simulink model "Y1_v2_v12"  (R2020a)
settings: Solver=VariableStepAuto  StartTime=0.0  StopTime=0.3  MaxStep=1e-5  RelTol=1e-3  EnableMultiTasking=on
libraries: simulink x1
settings Model: SimulationMode=accelerator  Creator=OXAALJ  LastModifiedBy=nxf75332
settings SolverCC: MaxOrder=2  MaxConsecutiveZCs=10  MaxConsecutiveMinStep=10  ZeroCrossControl=DisableAll
settings DataIOCC: LimitDataPoints=on  SaveFormat=Array  DSMLogging=off  ReturnWorkspaceOutputs=off
settings OptimizationCC: LifeSpan=inf
settings DebuggingCC: UnderspecifiedInitializationDetection=Classic  MergeDetectMultiDrivingBlocksExec=none  SolverPrmCheckMsg=warning  MultiTaskDSMMsg=warning  MultiTaskCondExecSysMsg=none  StateNameClashWarn=warning  SFUnexpectedBacktrackingDiag=warning  SFNoUnconditionalDefaultTransitionDiag=warning  SFExecutionAtInitializationDiag=none  ArithmeticOperatorsInVariantConditions=warning
settings HardwareCC: ProdBitPerPointer=32  ProdBitPerSizeT=32  ProdBitPerPtrDiffT=32  ProdLargestAtomicFloat=None  ProdIntDivRoundTo=Undefined  ProdEndianess=Unspecified  ProdWordSize=32  ProdHWDeviceType=32-bit Generic
settings ModelReferenceCC: PropagateSignalLabelsOutOfModel=off
settings SFSimCC: SimUseLocalCustomCode=off  CustomCodeUndefinedFunction=UseInterfaceOnly
settings RTWCC: RTWUseLocalCustomCode=off
settings CodeAppCC: StateflowObjectComments=on
settings GRTTargetCC: TargetLangStandard=C89/C90 (ANSI)
settings ConfigComp: CovMetricSettings=dw  CovHtmlReporting=on  CovSaveCumulativeToWorkspaceVar=on  CovSaveSingleToWorkspaceVar=on  CovExternalEMLEnable=off  CovSFcnEnable=off

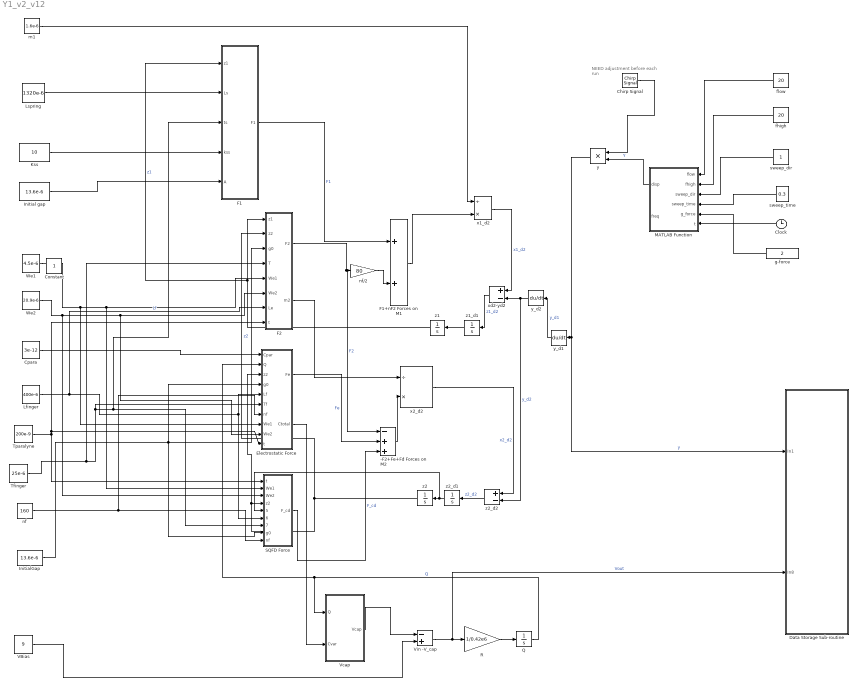
== system Y1_v2_v12 ==
  note: NEED
      | adjustment
      | before each
      | run
  -F2+Fe+Fd Forces on M2 : Sum  Inputs=-++  RndMeth=Nearest
  Chirp Signal : simulink/Sources/Chirp Signal  f1=20  T=0.3  f2=20
  Clock : Clock
  Cpara : Constant  Value=3e-12  VectorParams1D=off
  Data Storage Sub-routine : Subsystem
  Electrostatic Force : MATLAB Function  TreatAsAtomicUnit=on
  F1 : MATLAB Function  TreatAsAtomicUnit=on
  F1+nF2 Forces on M1 : Sum  RndMeth=Nearest
  F2 : MATLAB Function  TreatAsAtomicUnit=on
  Initial gap : Constant  Value=13.6e-6
  InitialGap : Constant  Value=13.6e-6
  Kss : Constant  Value=10
  Lfinger : Constant  Value=400e-6
  Lspring : Constant  Value=1320e-6
  MATLAB Function : MATLAB Function  TreatAsAtomicUnit=on
  Q : Integrator
  R : Gain  Gain=1/0.42e6
  SQFD Force : MATLAB Function  TreatAsAtomicUnit=on
  Tfinger : Constant  Value=25e-6
  Tparalyne : Constant  Value=200e-9  VectorParams1D=off
  VBias : Constant  Value=9
  Vcap : MATLAB Function  TreatAsAtomicUnit=on
  Vin -V_cap : Sum  Inputs=-+  RndMeth=Nearest
  We1 : Constant  Value=4.5e-6  VectorParams1D=off
  We2 : Constant  Value=20.9e-6  VectorParams1D=off
  fhigh : Constant  Value=20
  flow : Constant  Value=20
  g-force : Constant  Value=2
  m1 : Constant  Value=1.6e-6
  nf : Constant  Value=160
  nf/2 : Gain  Gain=80
  sweep_dir : Constant
  sweep_time : Constant  Value=0.3
  x1_d2 : Product  Inputs=/*
  x2_d2 : Product  Inputs=/*
  xd2-yd2 : Sum  Inputs=+-  RndMeth=Nearest
  y : Product
  y_d1 : Derivative
  y_d2 : Derivative
  z1 : Integrator
  z1_d1 : Integrator
  z2 : Integrator
  z2_d1 : Integrator
  z2_d2 : Sum  Inputs=+-  RndMeth=Nearest
  Constant : Constant  IOType=siggen
  wires:
  Electrostatic Force/1(Fe) -> -F2+Fe+Fd Forces on M2/2  "Fe"
  F1/1(F1) -> F1+nF2 Forces on M1/1  "F1"
  SQFD Force/1(F_cd) -> -F2+Fe+Fd Forces on M2/3  "F_cd"
  m1/1 -> x1_d2/1
  Clock/1 -> MATLAB Function/6(t)
  g-force/1 -> MATLAB Function/5(g_force)
  sweep_time/1 -> MATLAB Function/4(sweep_time)
  fhigh/1 -> MATLAB Function/2(fhigh)
  flow/1 -> MATLAB Function/1(flow)
  sweep_dir/1 -> MATLAB Function/3(sweep_dir)
  MATLAB Function/1(disp) -> y/2  "Y"
  y/1 -> Data Storage Sub-routine/1(In1), y_d1/1  "y"
  InitialGap/1 -> Electrostatic Force/4(g0), SQFD Force/8(g0), F2/3(g0)
  VBias/1 -> Vin -V_cap/2
  Vin -V_cap/1 -> Data Storage Sub-routine/2(In8), R/1  "Vout"
  R/1 -> Q/1
  Q/1 -> Electrostatic Force/2(Q), Vcap/1(Q)  "Q"
  Vcap/1(Vcap) -> Vin -V_cap/1
  Lfinger/1 -> F2/7(Le), Electrostatic Force/5(Lf), SQFD Force/6(Lf_damp)  "Lf"
  Cpara/1 -> Electrostatic Force/1(Cpar)
  Chirp Signal/1 -> y/1
  nf/1 -> Electrostatic Force/7(nf), SQFD Force/9(nf)
  Lspring/1 -> F1/2(Ls)
  Tfinger/1 -> F2/4(T), Electrostatic Force/6(Tf), F1/3(ts), SQFD Force/7(Tf_damp)
  Kss/1 -> F1/4(kss)
  F2/1(F2) -> -F2+Fe+Fd Forces on M2/1, nf/2/1  "F2"
  F1+nF2 Forces on M1/1 -> x1_d2/2
  y_d1/1 -> y_d2/1  "y_d1"
  x1_d2/1 -> xd2-yd2/1  "x1_d2"
  y_d2/1 -> z2_d2/2, xd2-yd2/2  "y_d2"
  xd2-yd2/1 -> z1_d1/1  "z1_d2"
  z1_d1/1 -> z1/1
  z1/1 -> F1/1(z1), F2/1(z1)  "z1"
  x2_d2/1 -> z2_d2/1  "x2_d2"
  z2_d2/1 -> z2_d1/1  "z2_d2"
  z2_d1/1 -> SQFD Force/5(z2_d1), z2/1
  z2/1 -> Electrostatic Force/3(z2), SQFD Force/4(z2), F2/2(z2)  "z2"
  F2/2(m2) -> x2_d2/1
  -F2+Fe+Fd Forces on M2/1 -> x2_d2/2
  nf/2/1 -> F1+nF2 Forces on M1/2
  Electrostatic Force/2(Ctotal) -> Vcap/2(Cvar)
  Initial gap/1 -> F1/5(A)
  We1/1 -> Electrostatic Force/8(We1), SQFD Force/2(We1), F2/5(We1)
  We2/1 -> SQFD Force/3(We2), Electrostatic Force/9(We2), F2/6(We2)
  Tparalyne/1 -> Electrostatic Force/10(t), F2/8(t), SQFD Force/1(t)

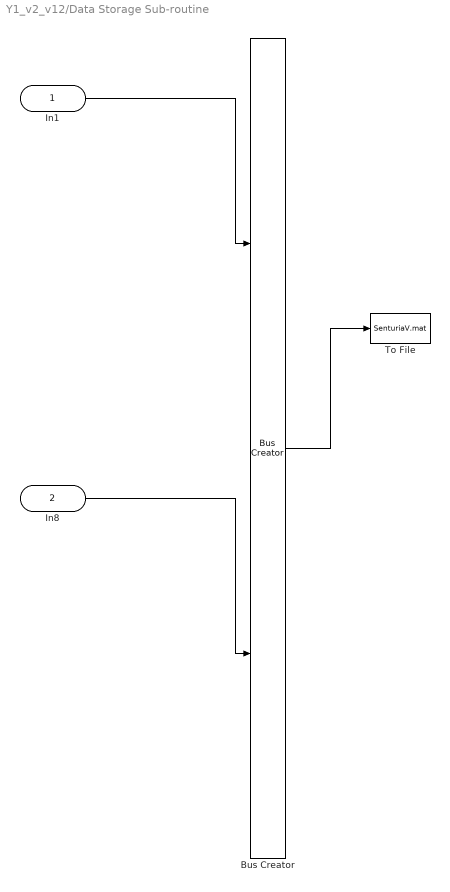
== system Y1_v2_v12/Data Storage Sub-routine ==
  In1 : Inport
  In8 : Inport  Port=2
  Bus Creator : BusCreator  Inputs=2
  To File : ToFile  Filename=SenturiaV.mat  SaveFormat=Timeseries
  wires:
  Bus Creator/1 -> To File/1
  In1/1 -> Bus Creator/1
  In8/1 -> Bus Creator/2

== matlab function Y1_v2_v12/Vcap ==
  data: Q input; Cvar input; Vcap output
function Vcap   = fcn(Q, Cvar)
Vcap = Q/Cvar;
end

== matlab function Y1_v2_v12/Electrostatic Force ==
  data: Cpar input; Q input; z2 input; g0 input; Lf input; Tf input; nf input; We1 input; Fe output; Ctotal output; We2 input; t input
function [Fe,Ctotal] = fcn(Cpar,Q,z2,g0,Lf,Tf,nf, We1, We2, t)
% This function is to calculate the Fe (electrostatic force on m2)

Lfeff =  Lf;
Tfeff =  Tf;
Lf    =  Tfeff;
Tf    =  Lfeff;


%%%% slanted electrodes (BASSET 2014)
a = (We2-We1)/2/Tf;    %aspect ratio
%C = ((eps0.*nf.*Lf)./(4.*a)).*log( ((g+2.*Wf.*a).^2 - z2.^2)./ (g.^2 - z2.^2));
% Cfit = (4.58916e18)*z2^6 - (6.34823e10)*z2^5 - (8.01379e8)*z2^4 + ...
%     (1.06902e1)*z2^3 + (8.85118e-2)*z2^2 + (3.66175e-11)*z2 + 1.50912e-11; % from excel
%Ctotal = Cfit + Cpar;
%==========================================================================
% Accounting for Parylene

eps0 = 8.85e-12;                                %permitivity of free space 
er   = 3.15;                                    %relative dielectric (Parylene C)
t    = 400e-9;                                  % thickness of parylene
g_p  = g0 - 2*t;                                % Minimum air gap
Ctot = 0;                                       % this gets reassigned in the if statements
z2lin = 1.54e-5;                              % z2 value at which linear approx starts
dcdz2 = 0.0605;                                % Slope of linear approx
c0 = 1.1855e-10;                                % Capacitance value at z2lin

if abs (z2) < g_p/2      %separate motion
    z2 = z2 * 2;
    C_L = ((eps0.*Lf)./(2.*a)).*( log( (g_p + z2 + 2.*a.*Tf)./(g_p + z2) ) );
    C_Leff = 1./( (2./(er.*eps0.*Lf.*Tf./t)) + 1./C_L);
    
    C_R = ((eps0.*Lf)./(2.*a)).*( log( (g_p - z2 + 2.*a.*Tf)./(g_p - z2) ) );
    C_Reff = 1 ./ ( (2./(er.*eps0.*Lf.*Tf./t)) + 1./C_R);

    Ctot = (C_Leff + C_Reff).*(nf./2);    
end

% if -z2lin > z2      % Impacting with Left Hand side
%     Ctot = c0 + dcdz2.*(-g_p - z2); 
% end 
% 
% if z2 > z2lin      % impacting with RHS
%     Ctot = c0 + dcdz2.*(z2 - g_p);
% end

Ctotal = Ctot + Cpar;
% z2max = 15.5e-6;     %maximum displaccement for capacitance calc
% Cmax = (4.58916e18)*z2max^6 - (6.34823e10)*z2max^5 - (8.01379e8)*z2max^4 + ...
%     (1.06902e1)*z2max^3 + (8.85118e-2)*z2max^2 + (3.66175e-11)*z2max...
%     + 1.50912e-11;      %capacitance at z2max
% C = min(Cmax,Cfit);     % Use Cmax if z2>z2max


% dC is divided by four here because nf is total electrodes, not number of
% electrode pairs
dC = ((eps0.*nf.*Lf)./(4.*a))*( ((2*z2)/(g0^2 - z2^2)) - ((2*z2)/((g0+2*Tf*a)^2 - z2^2) ));

% dC = ((eps0.*nf.*Lf)./(1*a))*( ((2*z2)/(g0^2 - z2^2)) - ((2*z2)/((g0+2*Tf*a)^2 - z2^2) ));  % Nf IS the number of electrodes

nFe = -1*((Q^2)/(2*Ctotal^2))*dC;

Fe = nFe./(nf/2);
end

== matlab function Y1_v2_v12/SQFD Force ==
  data: t input; We1 input; We2 input; z2 input; F_cd output; z2_d1 input; Lf_damp input; Tf_damp input; g0 input; nf input
function F_cd  = SQFD(t, We1, We2, z2,z2_d1,Lf_damp,Tf_damp,g0 ,nf)
% This block supports an embeddable subset of the MATLAB language.
% See the help menu for details. 
% 


mu = 1.846e-5;      %dynamic viscosity of air

%--------------------------------------------------------------------------
%Simple, low amplitude SQFD
% cd = nf*mu*Lf*Wf^3.*(1./(g-z).^3 + 1./(g+z).^3);
% A   = 14.4e-6;      %Soft Stopper Nominal Gap (meters)
% 
t    = 400e-9;                                  % thickness of parylene
g_p  = g0 - 2*t;                                % Minimum air gap


if  abs (z2) < g_p/2    %the separate motion
    z2 = 2*z2;
    z2_d1 = 2*z2_d1;
end   


%% Andy Moy damping Tf Lf
mu    =   1.983e-5*0.001;                                   %Air viscocity dynamic (kg/m*s)
rho   =   1.204;                                      %Air density    (kg/m3)                    
% a     =   (We2-We1)/Lf_damp;                          %Tilt angle difference, tan(a)- tan(b)
a     =   (We2-We1)/Lf_damp;                          %Tilt angle difference, tan(a)- tan(b)


t    = 200e-9;                                  % thickness of parylene
g_p  = g0 - 2*t;                                % Minimum air gap
% Left-hand side

ho_l  =  g_p + z2;                                    %Left-hand side ho
hl_l  =  ho_l + a*Lf_damp;                                %Left-hand side hl




C1_l  =  -ho_l*Lf_damp/(ho_l + 2*a)* z2_d1;               %The c1 parameter, left
C2_l  =  12*mu*a^-2/(2*ho_l + a*Lf_damp) * z2_d1;         %The c1 parameter, left


F_l   =  Tf_damp * (Lf_damp * C2_l - 6*mu*Lf_damp/a/ho_l/hl_l*C1_l + 6*mu*Lf_damp*a^-4/hl_l*z2_d1- 12*mu*a^-3 * z2_d1 * (log(ho_l./hl_l)) ); 
% F_l   =  Lf * (Tf * C2_l - 6*mu*Tf/a/ho_l/hl_l*C1_l + 6*mu*Tf*a^-4/hl_l*z2_d1+ 12*mu*a^-3 * z2_d1 * (log(16/22)) ); 
% Right-hand side                   

ho_r  =  g_p - z2;                                    %Left-hand side ho
hl_r  =  ho_r + a*Lf_damp;                                %Left-hand side hl

C1_r  =  -ho_r*Lf_damp/(ho_r + 2*a)* z2_d1;                 %The c1 parameter, right
C2_r  =  12*mu*a^-2/(2*ho_r + a*Lf_damp) * z2_d1;         %The c1 parameter, right

 
F_r   =  Tf_damp * (Lf_damp * C2_r - 6*mu*Lf_damp/a/ho_r/hl_r*C1_r + 6*mu*Lf_damp*a^-4/hl_r*z2_d1 + 12*mu*a^-3 * z2_d1 * (log(ho_r./hl_r) )) ; 

% nF_cd  =  -0.0010*(F_l  + F_r)*nf;
F_cd  =  -0.32*(F_l  + F_r);

end

== matlab function Y1_v2_v12/F2 ==
  data: z1 input; z2 input; F2 output; g0 input; m2 output; T input; We1 input; We2 input; Le input; t input
 function [F2, m2] = fcn(z1, z2, g0, T, We1, We2, Le, t)

%% Jinglun Li, lij31@rpi.edu/06/14/2019
% This is to calculate the F2 on m1 and m2, which is:

% Inputs:

% The displacement (z1)
% The displacement (z2)
% The effective spring constant k2 

% Output:
%  F2 = -k2 * (z1 - z2)

%% k2

E    =  180e9;                                   % The Young's mudulous 
t    =  400e-9;                                  % thickness of parylene
g_p  =  g0 - 2*t;                                % Minimum air gap
ro       = 2330;                                %Mass density               (kg/m3)
We_av    = mean([We1, We2]);                    %Electrode width (average)  (m)
Ie_r     =  1/12*T*We_av^3;

%% Force calculation
 if       abs (z2) < 0.5*g_p 
%           nm2      =    0.2e-8*(Nf/2);                     % Cantilever's mass
          m2       =    ro*T*Le*We_av;                       %Mass of single electrode
          k2       =    8*E/Le^3*Ie_r;                       %Spring constant of electrod
          F2       =   - k2*(z1 - z2);  
 else

%           nm2      =    0.2e-8;  
          m2       =    2*ro*T*Le*We_av ;                    % Cantilever's mass
          k2       =    8*E/Le^3*Ie_r;                       %Spring constant of electrode
          F2       =   - k2*(z1 - z2)+ k2*z2;                % From the second spring    
 end



end

== matlab function Y1_v2_v12/MATLAB Function ==
  data: flow input; disp output; fhigh input; sweep_dir input; sweep_time input; g_force input; t input; freq output
function [disp,freq] = fcn(flow,fhigh,sweep_dir,sweep_time,g_force,t)
%#codegen
% accel = g_force*9.81;

ramp = 200e-3;

if sweep_dir > 0
    %upsweep
    if t < ramp
        freq = (t/sweep_time)*(fhigh-flow) + flow;
        disp = (t/ramp)* (g_force/(4.0243*freq^2));          %const = (2*pi())^2/9.81
%         vel = (t/ramp)*(g_force*9.81)/(2*pi*freq);
    else
        freq = (t/sweep_time)*(fhigh-flow) + flow;
        disp = g_force/(4.0243*freq^2);          %const = (2*pi())^2/9.81
%         vel = (g_force*9.81)/(2*pi*freq);
%         disp = g/(4.0243*((fhigh-flow)/2)^2); 

%         freq = (0.5) * (fhigh+flow);
%         disp = g/(4.0243*freq^2);          %const = (2*pi())^2/9.81
    end
else
    %downsweep
    if t < ramp
        freq = fhigh - (t/sweep_time)*(fhigh-flow);
        disp = (t/ramp)* (g_force/(4.0243*freq^2));          %const = (2*pi())^2/9.81
%         vel = (t/ramp)*(g_force*9.81)/(2*pi*freq);
    else
        freq = fhigh - (t/sweep_time)*(fhigh-flow);
        disp = g_force/(4.0243*freq^2);          %const = (2*pi())^2/9.81
%         vel = (g_force*9.81)/(2*pi*freq);
%         disp = g/(4.0243*((fhigh-flow)/2)^2); 

%         freq = (0.5) * (fhigh+flow);
%         disp = g/(4.0243*freq^2);          %const = (2*pi())^2/9.81
    end
end
% freq = (t/sweep_time)*(fhigh-flow) + flow;
% freq = (0.5) * (fhigh+flow);
% disp = g/(4.0243*freq^2);          %const = (2*pi())^2/9.81
% disp = g/(4.0243*((fhigh-flow)/2)^2); 

% coder.extrinsic('chirp');
% y = chirp(t,flow,sweep_time,fhigh,'linear',0);
% y_dot = chirp(t,flow,sweep_time,fhigh,'linear',90);
% y_dot_dot = chirp(t,flow,sweep_time,fhigh,'linear',180);

end

== matlab function Y1_v2_v12/F1 ==
  data: z1 input; Ls input; ts input; kss input; A input; F1 output
function F1 = fcn(z1, Ls, ts, kss, A)

%% Jinglun Li, lij31@rpi.edu/06/14/2019
% This is to calculate the F1 on m1, which is:

% Inputs:
% The measuerd resonant frequency of m1
% The spring length of suspension spring
% The device thickness
% The spring constant of the softspring attache to the anchor
% The displacement (z11)


% Output:
%  F1 = Fsp +  Fss
%  Fsp - from the suspension spring
%  Fss - from the 


%% The device parameters, format should be constant ( all in SI unit)

E      =    180e9;                                   % The Young's mudulous 
ws     =    10e-6;                                   % spring width (m)


% k1       =    (omega0)^2*m1;                          %Linear spring constant k1 (N/m)
% wseff    = (((Ls^3)*k1)/(2*E*ts))^(1/3);         %effective spring beam width (m)
% k3_singu = (18/25)*(k1/2)*(1/(wseff^2));         %cubic spring constant of a single spring,  k3 (N/m)
% k3       = k3_singu/4;                           %k3 of all the connected suspension springs
% % 

k1      =    1/6*4*E *ts*(ws^3)/(Ls^3);                       % Spring constant from supporting beams
k3      =    1*(18/25)*E * ts*ws/(Ls^3);


%% Force calculation
% Fsp      =  -k1.*z1 - k3.*z1.^3;                 %Spring force from the suspension spring (N)
Fsp      =  -k1.*z1 - k3*1*(z1^3);                 %Spring force from the suspension spring (N)

%  Fss: to execute the piece-wise function

% To execute the piece-wise function
    if     abs (z1) < A
         Fss = 0;                                %No stoppers 
    else
         Fss = - kss*(z1-A)*sign(z1);          %Soft stopper
    end

F1       =   Fsp  +  Fss;                        %The spring force F1       


end
